simulink library "lowLevel"  (R2017b)
settings: Solver=VariableStepAuto  StartTime=0.0  StopTime=10.0  RelTol=1e-3
undefined symbols (not defined in the file): env, plant
libraries: lowLevel x1
settings Model: Creator=M.Cobb  LastModifiedBy=mitch
settings CodeAppCC: StateflowObjectComments=on

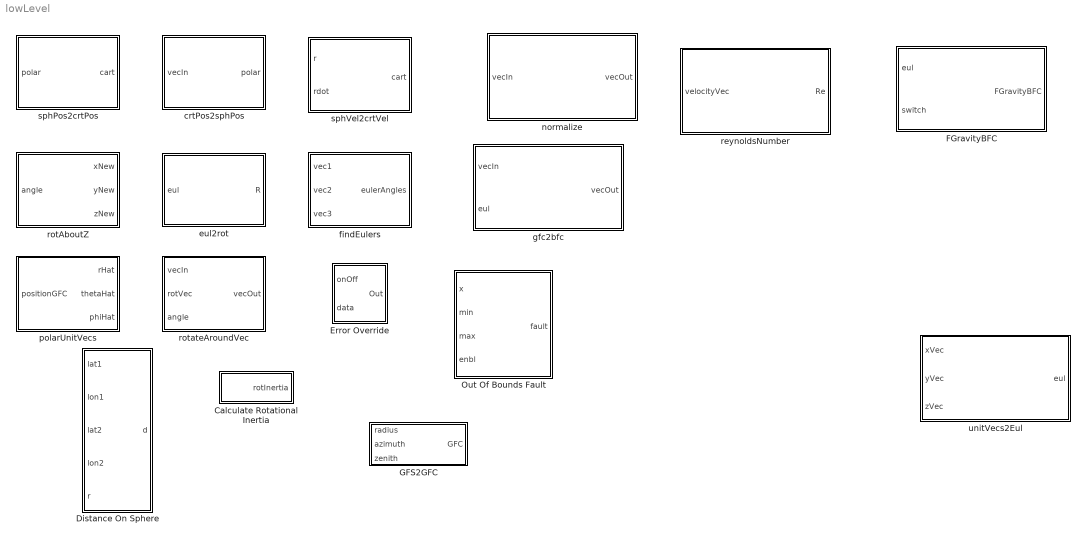
== system lowLevel ==
  Calculate Rotational Inertia : Subsystem
  Distance On Sphere : Subsystem
  Error Override : Subsystem
  FGravityBFC : Subsystem
  GFS2GFC : Subsystem
  Out Of Bounds Fault : Subsystem
  crtPos2sphPos : MATLAB Function  TreatAsAtomicUnit=on
  eul2rot : MATLAB Function  TreatAsAtomicUnit=on
  findEulers : MATLAB Function  TreatAsAtomicUnit=on
  gfc2bfc : Subsystem
  normalize : Subsystem
  polarUnitVecs : MATLAB Function  TreatAsAtomicUnit=on
  reynoldsNumber : Subsystem
  rotAboutZ : MATLAB Function  TreatAsAtomicUnit=on
  rotateAroundVec : MATLAB Function  TreatAsAtomicUnit=on
  sphPos2crtPos : MATLAB Function  TreatAsAtomicUnit=on
  sphVel2crtVel : MATLAB Function  TreatAsAtomicUnit=on
  unitVecs2Eul : Subsystem

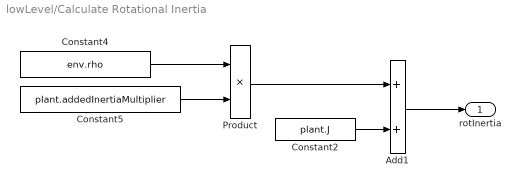
== system lowLevel/Calculate Rotational Inertia ==
  Add1 : Sum
  Constant2 : Constant  Value=plant.J
  Constant4 : Constant  Value=env.rho
  Constant5 : Constant  Value=plant.addedInertiaMultiplier
  Product : Product
  rotInertia : Outport
  wires:
  Constant4/1 -> Product/1
  Add1/1 -> rotInertia/1
  Constant2/1 -> Add1/2
  Product/1 -> Add1/1
  Constant5/1 -> Product/2

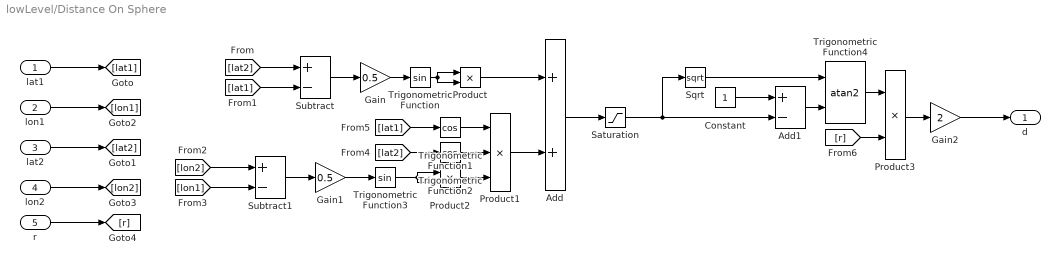
== system lowLevel/Distance On Sphere ==
  lat1 : Inport
  lon1 : Inport  Port=2
  lat2 : Inport  Port=3
  lon2 : Inport  Port=4
  r : Inport  Port=5
  Add : Sum
  Add1 : Sum  Inputs=+-
  Constant : Constant
  Gain : Gain  Gain=0.5
  Gain1 : Gain  Gain=0.5
  Gain2 : Gain  Gain=2
  Product : Product
  Product1 : Product  Inputs=3
  Product2 : Product
  Product3 : Product
  Saturation : Saturate  UpperLimit=1  LowerLimit=0
  Sqrt : Sqrt  SaturateOnIntegerOverflow=on
  Subtract : Sum  Inputs=+-
  Subtract1 : Sum  Inputs=+-
  Trigonometric Function : Trigonometry
  Trigonometric Function1 : Trigonometry  Operator=cos
  Trigonometric Function2 : Trigonometry  Operator=cos
  Trigonometric Function3 : Trigonometry
  Trigonometric Function4 : Trigonometry  Operator=atan2
  d : Outport
  wires:
  Gain/1 -> Trigonometric Function/1
  Subtract/1 -> Gain/1
  Trigonometric Function/1 -> Product/2, Product/1
  Subtract1/1 -> Gain1/1
  [lon1] -> Subtract1/2
  [lon2] -> Subtract1/1
  Sqrt/1 -> Trigonometric Function4/1
  Trigonometric Function1/1 -> Product1/1
  Trigonometric Function4/1 -> Product3/1
  Product/1 -> Add/1
  [r] -> Product3/2
  Constant/1 -> Add1/1
  [lat1] -> Subtract/2
  Product1/1 -> Add/2
  Trigonometric Function2/1 -> Product1/2
  Add/1 -> Saturation/1
  Add1/1 -> Trigonometric Function4/2
  Product3/1 -> Gain2/1
  [lat1] -> Trigonometric Function1/1
  [lat2] -> Trigonometric Function2/1
  Product2/1 -> Product1/3
  [lat2] -> Subtract/1
  Saturation/1 -> Add1/2, Sqrt/1
  Trigonometric Function3/1 -> Product2/2, Product2/1
  Gain2/1 -> d/1
  Gain1/1 -> Trigonometric Function3/1
  lon1/1 -> [lon1]
  lat1/1 -> [lat1]
  lat2/1 -> [lat2]
  lon2/1 -> [lon2]
  r/1 -> [r]

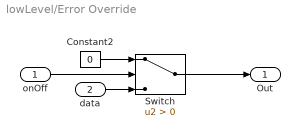
== system lowLevel/Error Override ==
  onOff : Inport
  data : Inport  Port=2
  Constant2 : Constant  Value=0
  Switch : Switch  Criteria=u2 > Threshold
  Out : Outport
  wires:
  Switch/1 -> Out/1
  onOff/1 -> Switch/2
  Constant2/1 -> Switch/1
  data/1 -> Switch/3

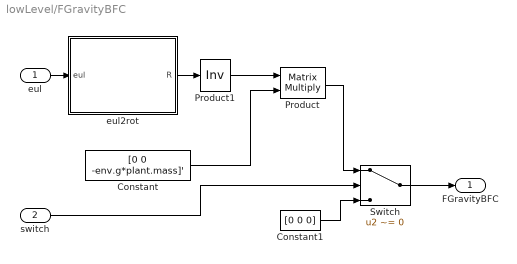
== system lowLevel/FGravityBFC ==
  eul : Inport
  switch : Inport  Port=2
  Constant : Constant  Value=[0 0 -env.g*plant.mass]'
  Constant1 : Constant  Value=[0 0 0]
  Product : Product  Multiplication=Matrix(*)
  Product1 : Product  Inputs=/  Multiplication=Matrix(*)
  Switch : Switch  Criteria=u2 ~= 0
  eul2rot : MATLAB Function  TreatAsAtomicUnit=on
  FGravityBFC : Outport
  wires:
  eul2rot/1(R) -> Product1/1
  eul/1 -> eul2rot/1(eul)
  Constant1/1 -> Switch/3
  switch/1 -> Switch/2
  Product/1 -> Switch/1
  Switch/1 -> FGravityBFC/1
  Product1/1 -> Product/1
  Constant/1 -> Product/2

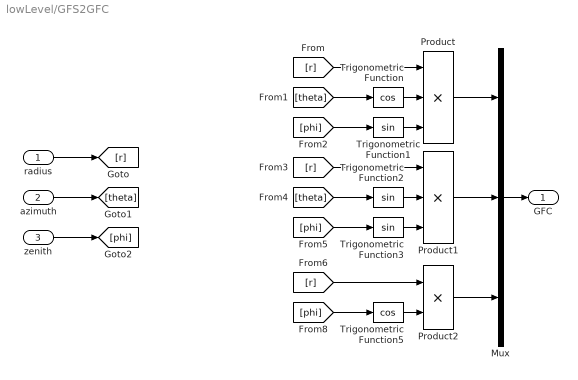
== system lowLevel/GFS2GFC ==
  radius : Inport
  azimuth : Inport  Port=2
  "zenith " : Inport  Port=3
  Mux : Mux  Inputs=3
  Product : Product  Inputs=3
  Product1 : Product  Inputs=3
  Product2 : Product
  Trigonometric Function : Trigonometry  Operator=cos
  Trigonometric Function1 : Trigonometry
  Trigonometric Function2 : Trigonometry
  Trigonometric Function3 : Trigonometry
  Trigonometric Function5 : Trigonometry  Operator=cos
  GFC : Outport
  wires:
  radius/1 -> [r]
  azimuth/1 -> [theta]
  "zenith "/1 -> [phi]
  Mux/1 -> GFC/1
  Product/1 -> Mux/1
  [r] -> Product/1
  Trigonometric Function/1 -> Product/2
  Trigonometric Function1/1 -> Product/3
  [phi] -> Trigonometric Function1/1
  [theta] -> Trigonometric Function/1
  [theta] -> Trigonometric Function2/1
  Trigonometric Function2/1 -> Product1/2
  Trigonometric Function3/1 -> Product1/3
  [r] -> Product1/1
  [phi] -> Trigonometric Function3/1
  Product1/1 -> Mux/2
  [r] -> Product2/1
  [phi] -> Trigonometric Function5/1
  Product2/1 -> Mux/3
  Trigonometric Function5/1 -> Product2/2

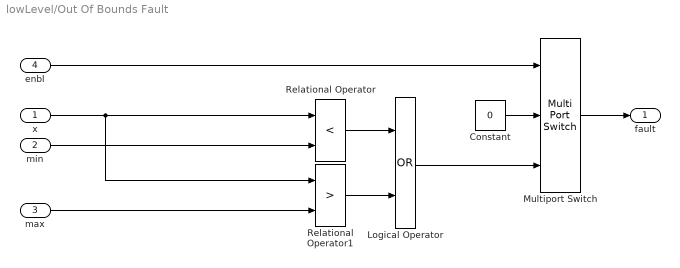
== system lowLevel/Out Of Bounds Fault ==
  x : Inport
  min : Inport  Port=2
  max : Inport  Port=3
  enbl : Inport  Port=4
  Constant : Constant  Value=0  OutDataTypeStr=boolean
  Logical Operator : Logic  Operator=OR  AllPortsSameDT=off  OutDataTypeStr=boolean
  Multiport Switch : MultiPortSwitch  DataPortOrder=Zero-based contiguous  Inputs=2
  Relational Operator : RelationalOperator  Operator=<  OutDataTypeStr=boolean  RndMeth=Simplest
  Relational Operator1 : RelationalOperator  Operator=>  OutDataTypeStr=boolean  RndMeth=Simplest
  fault : Outport
  wires:
  Relational Operator/1 -> Logical Operator/1
  Relational Operator1/1 -> Logical Operator/2
  min/1 -> Relational Operator/2
  x/1 -> Relational Operator1/1, Relational Operator/1
  max/1 -> Relational Operator1/2
  Multiport Switch/1 -> fault/1
  enbl/1 -> Multiport Switch/1
  Logical Operator/1 -> Multiport Switch/3
  Constant/1 -> Multiport Switch/2

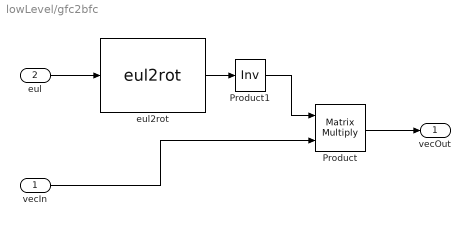
== system lowLevel/gfc2bfc ==
  vecIn : Inport
  eul : Inport  Port=2
  Product : Product  Multiplication=Matrix(*)
  Product1 : Product  Inputs=/  Multiplication=Matrix(*)
  eul2rot : lowLevel/eul2rot
  vecOut : Outport
  wires:
  Product1/1 -> Product/1
  eul2rot/1 -> Product1/1
  eul/1 -> eul2rot/1
  vecIn/1 -> Product/2
  Product/1 -> vecOut/1

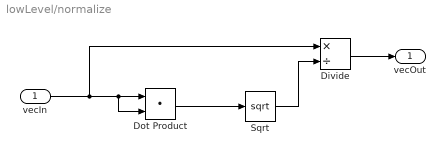
== system lowLevel/normalize ==
  vecIn : Inport
  Divide : Product  Inputs=*/
  Dot Product : DotProduct  InputSameDT=on  OutDataTypeStr=Inherit: Inherit via internal rule
  Sqrt : Sqrt  SaturateOnIntegerOverflow=on
  vecOut : Outport
  wires:
  vecIn/1 -> Divide/1, Dot Product/2, Dot Product/1
  Dot Product/1 -> Sqrt/1
  Sqrt/1 -> Divide/2
  Divide/1 -> vecOut/1

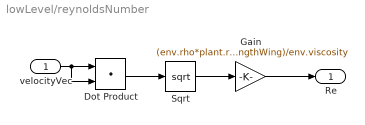
== system lowLevel/reynoldsNumber ==
  velocityVec : Inport
  Dot Product : DotProduct  InputSameDT=on  OutDataTypeStr=Inherit: Inherit via internal rule
  Gain : Gain  Gain=(env.rho*plant.refLengthWing)/env.viscosity
  Sqrt : Sqrt  SaturateOnIntegerOverflow=on
  Re : Outport
  wires:
  Gain/1 -> Re/1
  velocityVec/1 -> Dot Product/2, Dot Product/1
  Dot Product/1 -> Sqrt/1
  Sqrt/1 -> Gain/1

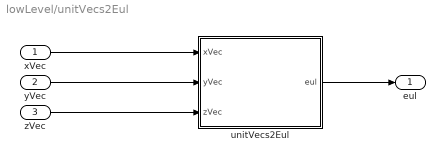
== system lowLevel/unitVecs2Eul ==
  xVec : Inport
  yVec : Inport  Port=2
  zVec : Inport  Port=3
  unitVecs2Eul : MATLAB Function  TreatAsAtomicUnit=on
  eul : Outport
  wires:
  xVec/1 -> unitVecs2Eul/1(xVec)
  yVec/1 -> unitVecs2Eul/2(yVec)
  zVec/1 -> unitVecs2Eul/3(zVec)
  unitVecs2Eul/1(eul) -> eul/1

== matlab function lowLevel/sphVel2crtVel ==
  data: r input; cart output; rdot input
function cart = sphVel2crtVel(r,rdot)
% convert a ground fixed polar vector to ground fixed cartesian
% This follows the wolfram convention outlined here:
% http://mathworld.wolfram.com/SphericalCoordinates.html
cart = [0;0;0];
cart(1) =       cos(r(2))*sin(r(3))*rdot(1)...
          -r(1)*sin(r(2))*sin(r(3))*rdot(2)...
          +r(1)*cos(r(2))*cos(r(3))*rdot(3);

cart(2) =       sin(r(2))*sin(r(3))*rdot(1)...
          +r(1)*cos(r(2))*sin(r(3))*rdot(2)...
          +r(1)*sin(r(2))*cos(r(3))*rdot(3);

cart(3) = cos(r(3))*rdot(1)-r(1)*sin(r(3))*rdot(3);
end

== matlab function lowLevel/eul2rot ==
  data: eul input; R output
function R = eul2rot(eul)
% Convert Euler angles to rotation Matrix
ct = cos(eul);
st = sin(eul);

%     The rotation matrix R can be constructed as follows by
%     ct = [cz cy cx] and st = [sy sy sx]
%
%     R = [  cy*cz   sy*sx*cz-sz*cx    sy*cx*cz+sz*sx
%            cy*sz   sy*sx*sz+cz*cx    sy*cx*sz-cz*sx
%              -sy            cy*sx             cy*cx]
%       = Rz(tz) * Ry(ty) * Rx(tx)
R=zeros(3,3);
R(1,1) = ct(2).*ct(1);
R(1,2) = st(3).*st(2).*ct(1) - ct(3).*st(1);
R(1,3) = ct(3).*st(2).*ct(1) + st(3).*st(1);
R(2,1) = ct(2).*st(1);
R(2,2) = st(3).*st(2).*st(1) + ct(3).*ct(1);
R(2,3) = ct(3).*st(2).*st(1) - st(3).*ct(1);
R(3,1) = -st(2);
R(3,2) = st(3).*ct(2);
R(3,3) = ct(3).*ct(2);
        
        
end

== matlab function lowLevel/FGravityBFC/eul2rot ==
  data: eul input; R output
function R = eul2rot(eul)
% Convert Euler angles to rotation Matrix
ct = cos(eul);
st = sin(eul);

%     The rotation matrix R can be constructed as follows by
%     ct = [cz cy cx] and st = [sy sy sx]
%
%     R = [  cy*cz   sy*sx*cz-sz*cx    sy*cx*cz+sz*sx
%            cy*sz   sy*sx*sz+cz*cx    sy*cx*sz-cz*sx
%              -sy            cy*sx             cy*cx]
%       = Rz(tz) * Ry(ty) * Rx(tx)
R=zeros(3,3);
R(1,1) = ct(2).*ct(1);
R(1,2) = st(3).*st(2).*ct(1) - ct(3).*st(1);
R(1,3) = ct(3).*st(2).*ct(1) + st(3).*st(1);
R(2,1) = ct(2).*st(1);
R(2,2) = st(3).*st(2).*st(1) + ct(3).*ct(1);
R(2,3) = ct(3).*st(2).*st(1) - st(3).*ct(1);
R(3,1) = -st(2);
R(3,2) = st(3).*ct(2);
R(3,3) = ct(3).*ct(2);
        
        
end

== matlab function lowLevel/crtPos2sphPos ==
  data: vecIn input; polar output
function polar = cart2sphere(vecIn)
% convert a cartesian vector to a spherical vector
% this follows the conventioned outlined here: 
% http://mathworld.wolfram.com/SphericalCoordinates.html
polar = [0;0;0];
% polar(1) = sqrt(sum(cart.^2));
% polar(2) = atan2(cart(2),cart(1));
% polar(3) = (pi/2)-acos(cart(3)/polar(1));
polar(1) = sqrt(sum(vecIn.^2));         %r
polar(2) = atan2(vecIn(2),vecIn(1));    %theta
polar(3) = acos(vecIn(3)/polar(1));            %phi
end

== matlab function lowLevel/sphPos2crtPos ==
  data: polar input; cart output
function cart = sphere2cart(polar)
% convert a ground fixed polar vector to ground fixed cartesian
% This follows the wolfram convention outlined here:
% http://mathworld.wolfram.com/SphericalCoordinates.html
cart = [0;0;0];
cart(1) = polar(1)*cos(polar(2))*sin(polar(3));
cart(2) = polar(1)*sin(polar(2))*sin(polar(3));
cart(3) = polar(1)*cos(polar(3));
end

== matlab function lowLevel/polarUnitVecs ==
  data: positionGFC input; rHat output; thetaHat output; phiHat output
function [rHat,thetaHat,phiHat] = polarUnitVecs(positionGFC)
% Find ground-frame representation of spherical unit vectors for a given
% cartesian vector.  Each unit vector output is represented in ground frame
% cartesian components This follows the wolfram convention outlined here:
% http://mathworld.wolfram.com/SphericalCoordinates.html
r       = sqrt(sum(positionGFC.^2));
theta   = atan2(positionGFC(2),positionGFC(1));
phi     = acos(positionGFC(3)/r);

rHat        = [cos(theta)*sin(phi)  sin(theta)*sin(phi) cos(phi)    ]';
thetaHat    = [-sin(theta)          cos(theta)          0           ]';
phiHat      = [cos(theta)*cos(phi)  sin(theta)*cos(phi) -sin(phi)   ]';
end

== matlab function lowLevel/rotAboutZ ==
  data: angle input; xNew output; yNew output; zNew output
function [xNew,yNew,zNew] = rotAboutZ(angle)
% Function takes the body fixed x, y, anz axes and rotates them about the z
% axis by the amount specified in angle.
xHat = [1 0 0]';
yHat = [0 1 0]';
zHat = [0 0 1]';
R = [cos(angle),-sin(angle) 0;sin(angle) cos(angle) 0;0 0 1];
xNew = R*xHat;
yNew = R*yHat;
zNew = R*zHat;

end

== matlab function lowLevel/findEulers ==
  data: vec1 input; eulerAngles output; vec2 input; vec3 input
function eulerAngles = findEulers(vec1,vec2,vec3)
% Function takes the sperical thetaHat and phiHat and rotates about the
% rHat vector by the amount specified in angle.  Returns 3 3-element column
% vectors representing the new vectors in spherical coordinates.
rHat = [1 0 0]';
thetaHat = [0 1 0]';
phiHat = [0 0 1]';
rot = [cos(angle) -sin(angle) 0; sin(angle) cos(angle) 0;0 0 1];
rNew = rot*rHat;
thetaNew = rot*thetaHat;
phiNew = rot*phiHat;
end

== matlab function lowLevel/rotateAroundVec ==
  data: vecIn input; vecOut output; rotVec input; angle input
function vecOut = rotateAroundVec(vecIn,rotVec,angle)
% Function rotates a vector around an arbitrary vector.
% vecIn = vector to be rotated
% rotVec = vector that defines the axis of rotation
% angle = the angle of rotation
% vecOut = angle after rotation
% This follows the procedure outlined here:
% http://ksuweb.kennesaw.edu/~plaval//math4490/rotgen.pdf
% position=vecIn';
% T=[1 0 0 -position(1);0 1 0 -position(2);0 0 1 -position(3);0 0 0 1];
% Tinv=[1 0 0 position(1);0 1 0 position(2);0 0 1 position(3);0 0 0 1];
% vecIn = [vecIn(1) vecIn(2) vecIn(3) 1]./sqrt(sum(vecIn.^2));
% vecOut = zeros(3,1);
% a = rotVec(1);
% b = rotVec(2);
% c = rotVec(3);
% d = sqrt(b^2+c^2);
% if d~=0
%     Rx = [1 0 0 0;0 c/d -b/d 0;0 b/d c/d 0;0 0 0 1];
%     RxInv = Rx';
%     Ry = [d 0 -a 0;0 1 0 0;a 0 d 0;0 0 0 1];
%     RyInv = Ry';
%     Rz=[cos(angle) -sin(angle) 0 0;sin(angle) cos(angle) 0 0;0 0 1 0;0 0 0 1];
%     vec = Tinv*RxInv*RyInv*Rz*Ry*Rx*T*vecIn';
%     vecOut = [vec(1) vec(2) vec(3)]';
% else
%     vecOut = position';
% end

C=cos(angle);
S=sin(angle);
t=1-cos(angle);
r=rotVec./sqrt(sum(rotVec.^2));
ux=r(1);uy=r(2);uz=r(3);
R=[t*ux^2+C        t*ux*uy-S*uz    t*ux*uz+S*uy;...
   t*ux*uy+S*uz    t*uy^2+C        t*uy*uz-S*ux;...
   t*ux*uz-S*uy    t*uy*uz+S*ux    t*uz^2+C];
vecOutTranspose = R*[vecIn(1);vecIn(2);vecIn(3)];
vecOut = vecOutTranspose';
end

== matlab function lowLevel/unitVecs2Eul/unitVecs2Eul ==
  data: xVec input; eul output; yVec input; zVec input
function eul = unitVecs2Eul(xVec,yVec,zVec)
% Function to convert unit vectors to euler angles
% Adapted from http://citeseerx.ist.psu.edu/viewdoc/download?doi=10.1.1.371.6578&rep=rep1&type=pdf
R=[xVec(1) yVec(1) zVec(1);xVec(2) yVec(2) zVec(2);xVec(3) yVec(3) zVec(3)];
eul = zeros(1,3);

%For a given matrix R, there are two sets of possible values for eul
%This provides the first one
if (R(3,1)~=1)&&(R(3,1)~=-1)
    eul(2) = -asin(R(3,1));
    eul(3) = atan2(R(3,2)/cos(eul(2)),R(3,3)/cos(eul(2)));
    eul(1) = atan2(R(2,1)/cos(eul(2)),R(1,1)/cos(eul(2)));
else
    eul(1) = 0;
    if R(3,1)==-1
        eul(2) = pi/2;
        eul(3) = atan2(R(1,2),R(1,3));
    else
        eul(2) = -pi/2;
        eul(3) = atan2(-R(1,2),R(1,3));
    end
end
end
